simulink model "SimulinkCarre"  (R2016a)
settings: Solver=VariableStepAuto  StartTime=0.0  StopTime=4*Tsim  RelTol=1e-3
values from neighbouring files (symbols this model uses):
  F0 = 85000    [Script.m]
  Te = 1/320000    (= 3.125e-06)    [Script.m]    (also in matlab1.mat = 0.03125; test.m = 1/M)
  Ts = Te/100    (= 3.125e-08)    [Script.m]    (also in matlab1.mat = 0.0003125; test.m = Te/100)
settings Model: Creator=ferrandi  LastModifiedBy=ferrandi

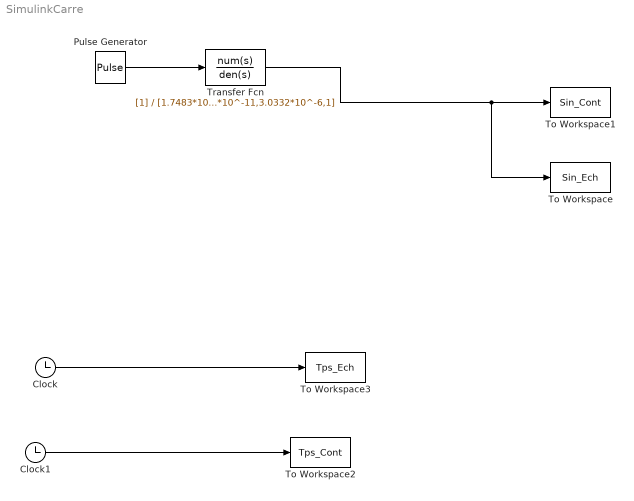
== system SimulinkCarre ==
  Clock : Clock
  Clock1 : Clock
  Pulse Generator : DiscretePulseGenerator  PulseType=Time based  Period=1/F0  PulseWidth=50
  To Workspace : ToWorkspace  VariableName=Sin_Ech  SaveFormat=Timeseries  SampleTime=Te
  To Workspace1 : ToWorkspace  VariableName=Sin_Cont  SaveFormat=Timeseries  SampleTime=Ts
  To Workspace2 : ToWorkspace  VariableName=Tps_Cont  SaveFormat=Timeseries  SampleTime=Ts
  To Workspace3 : ToWorkspace  VariableName=Tps_Ech  SaveFormat=Timeseries  SampleTime=Te
  Transfer Fcn : TransferFcn  Denominator=[1.7483*10^-23,7.6663*10^-18,1.162*10^-11,3.0332*10^-6,1]
  wires:
  Clock1/1 -> To Workspace2/1
  Clock/1 -> To Workspace3/1
  Pulse Generator/1 -> Transfer Fcn/1
  Transfer Fcn/1 -> To Workspace/1, To Workspace1/1
